simulink model "kalman"  (R2015a)
settings: Solver=ode45  StartTime=0.0  StopTime=500  RelTol=1e-3
settings Model: Creator=ry0  LastModifiedBy=ry0

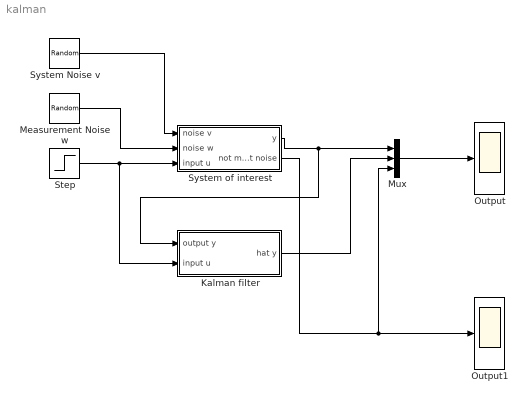
== system kalman ==
  Kalman filter : Subsystem
  Measurement Noise w : RandomNumber  Variance=0.7  SampleTime=0.1
  Mux : Mux  Inputs=3
  Output : Scope
      settings: YMin=-10  YMax=80  SaveName=ScopeData3
  Output1 : Scope
      settings: YMin=-10  YMax=80
  Step : Step  After=1000  SampleTime=0
  System Noise v : RandomNumber  Variance=0.7  Seed=1  SampleTime=0.1
  System of interest : Subsystem
  wires:
  Kalman filter/1(hat y) -> Mux/2
  Measurement Noise w/1 -> System of interest/2(noise w)
  System Noise v/1 -> System of interest/1(noise v)
  Step/1 -> Kalman filter/2("input u "), System of interest/3("input u ")
  System of interest/1(y) -> Kalman filter/1(output y), Mux/1
  Mux/1 -> Output/1
  System of interest/2("not measurement noise ") -> Mux/3, Output1/1

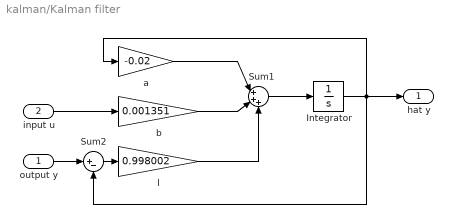
== system kalman/Kalman filter ==
  output y : Inport
  "input u " : Inport  Port=2
  Integrator : Integrator
  Sum1 : Sum  Inputs=|+++
  Sum2 : Sum  Inputs=|+-
  a : Gain  Gain=-0.02
  b : Gain  Gain=0.001351
  l : Gain  Gain=0.998002
  hat y : Outport
  wires:
  output y/1 -> Sum2/1
  "input u "/1 -> b/1
  Sum1/1 -> Integrator/1
  Integrator/1 -> a/1, Sum2/2, hat y/1
  Sum2/1 -> l/1
  a/1 -> Sum1/1
  b/1 -> Sum1/2
  l/1 -> Sum1/3

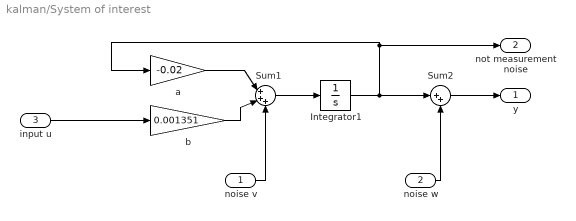
== system kalman/System of interest ==
  noise v : Inport
  noise w : Inport  Port=2
  "input u " : Inport  Port=3
  Integrator1 : Integrator
  Sum1 : Sum  Inputs=|+++
  Sum2 : Sum  Inputs=|++
  a : Gain  Gain=-0.02
  b : Gain  Gain=0.001351
  y : Outport
  "not measurement noise " : Outport  Port=2
  wires:
  noise v/1 -> Sum1/3
  Sum2/1 -> y/1
  noise w/1 -> Sum2/2
  "input u "/1 -> b/1
  Sum1/1 -> Integrator1/1
  Integrator1/1 -> "not measurement noise "/1, a/1, Sum2/1
  a/1 -> Sum1/1
  b/1 -> Sum1/2
